simulink model "simTrue"  (R2020a)
settings: Solver=ode3  StartTime=0.0  StopTime=simPrm.tEnd  FixedStep=simPrm.dt  RelTol=1e-3
values from neighbouring files (symbols this model uses):
  A = [ 0    0        1     0 ... (first row only)    [setupTrue.m]
  B = [0;0;Mat.B31;Mat.B41]    [setupTrue.m]
  C = [1 0 0 0 ... (first row only)    [setupTrue.m]
  D = [0;0;0;0]    [setupTrue.m]
  V = 1    [setupTrue.m]
undefined symbols (not defined in the file or in its folder): Input
settings Model: Creator=vmali  LastModifiedBy=vmali

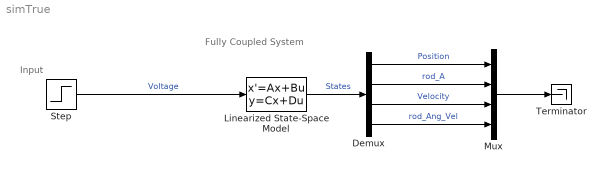
== system simTrue ==
  note: Fully Coupled System
  note: Input
  Demux : Demux
  Linearized State-Space Model : StateSpace  A=A  B=B  C=C  D=D  InitialCondition=0
  Mux : Mux
  Step : Step  Time=Input.ts  After=V  SampleTime=0
      settings: AttributesFormatString=%<After>
  Terminator : Terminator
  wires:
  Step/1 -> Linearized State-Space Model/1  "Voltage"
  Linearized State-Space Model/1 -> Demux/1  "States"
  Mux/1 -> Terminator/1
  Demux/1 -> Mux/1  "Position"
  Demux/2 -> Mux/2  "rod_A"
  Demux/3 -> Mux/3  "Velocity"
  Demux/4 -> Mux/4  "rod_Ang_Vel"
